simulink model "fzy_simulation"  (R2014b)
settings: Solver=ode3  StartTime=0.0  StopTime=5  FixedStep=0.001  RelTol=1e-3
libraries: fuzblock x1
settings Model: Creator=nk  LastModifiedBy=nk

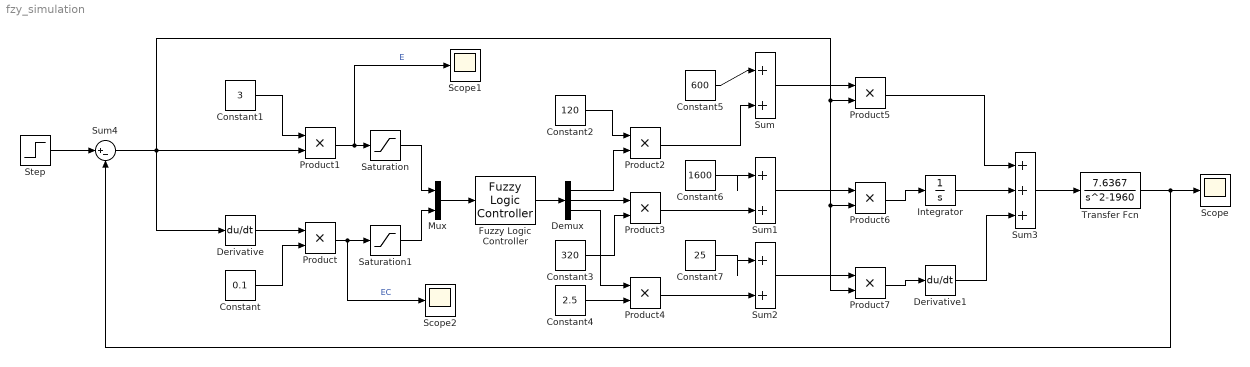
== system fzy_simulation ==
  Constant : Constant  Value=0.1
  Constant1 : Constant  Value=3
  Constant2 : Constant  Value=120
  Constant3 : Constant  Value=320
  Constant4 : Constant  Value=2.5
  Constant5 : Constant  Value=600
  Constant6 : Constant  Value=1600
  Constant7 : Constant  Value=25
  Demux : Demux  Outputs=3
  Derivative : Derivative
  Derivative1 : Derivative
  Fuzzy Logic Controller : fuzblock/Fuzzy Logic  Controller  fis=fzy
  Integrator : Integrator
  Mux : Mux  Inputs=2
  Product{,1..7} (8 alike) : Product
  Saturation : Saturate
  Saturation1 : Saturate
  Scope : Scope
      settings: YMin=0  YMax=2  SaveName=FZY  MaxDataPoints=500000000
  Scope1 : Scope
  Scope2 : Scope
  Step : Step  SampleTime=0
  Sum : Sum  Inputs=|++
  Sum1 : Sum  Inputs=|++
  Sum2 : Sum  Inputs=|++
  Sum3 : Sum  Inputs=+++
  Sum4 : Sum  Inputs=|+-
  Transfer Fcn : TransferFcn  Numerator=[7.6367]  Denominator=[1 0 -1960]
  wires:
  Constant1/1 -> Product1/1
  Sum4/1 -> Derivative/1, Product7/2, Product6/2, Product5/2, Product1/2
  Derivative/1 -> Product/1
  Constant/1 -> Product/2
  Product1/1 -> Scope1/1, Saturation/1  "E"
  Product/1 -> Scope2/1, Saturation1/1  "EC"
  Saturation/1 -> Mux/1
  Saturation1/1 -> Mux/2
  Mux/1 -> Fuzzy Logic Controller/1
  Fuzzy Logic Controller/1 -> Demux/1
  Demux/1 -> Product2/2
  Demux/2 -> Product3/1
  Demux/3 -> Product4/1
  Constant2/1 -> Product2/1
  Constant3/1 -> Product3/2
  Constant4/1 -> Product4/2
  Constant5/1 -> Sum/1
  Product2/1 -> Sum/2
  Constant6/1 -> Sum1/1
  Product3/1 -> Sum1/2
  Constant7/1 -> Sum2/1
  Product4/1 -> Sum2/2
  Sum/1 -> Product5/1
  Sum1/1 -> Product6/1
  Sum2/1 -> Product7/1
  Product5/1 -> Sum3/1
  Product6/1 -> Integrator/1
  Integrator/1 -> Sum3/2
  Product7/1 -> Derivative1/1
  Derivative1/1 -> Sum3/3
  Step/1 -> Sum4/1
  Sum3/1 -> Transfer Fcn/1
  Transfer Fcn/1 -> Sum4/2, Scope/1
